simulink model "SimParking"  (R2017b)
settings: Solver=VariableStepAuto  StartTime=0.0  StopTime=1761  RelTol=1e-3
libraries: neural x1111
(part 40 of 60)

== system SimParking/BestNet- 10 delays -100 100 hidden neurons/Layer 3/Delays 1 ==
  "p{3}" : Inport  PortDimensions=100  SampleTime=1
      mask Display: e = 0.06;c1 = [120 230 180]/255;c2 = ([120 230 180]+0)/(256+128);c3 = ([120 230 180]+128)/(256+128);patch([0 1 1 0],[0 0 1 1],c1);patch([0 1 1 1-e 1-e 0+e],[0 0 1 1-e 0+e 0+e],c2);patch([0 0 1 1-e 0+e 0+e],[0 1 1 1-e 1-e 0+e],c3);plot([0 1 1 0 0],[0 0 1 1 0]);
  mux : Mux  Inputs=1
      mask Display: e = 0.06;c1 = [120 150 230]/255;c2 = ([120 150 230]+0)/383;c3 = ([120 150 230]+128)/383;patch([0 1 1 0],[0 0 1 1],c1);patch([0 1 1 1-e 1-e 0+e],[0 0 1 1-e 0+e 0+e],c2);patch([0 0 1 1-e 0+e 0+e],[0 1 1 1-e 1-e 0+e],c3);plot([0 1 1 0 0],[0 0 1 1 0]);disp('Mux')
  "pd{3,2}" : Outport
      mask Display: e = 0.06;c1 = [120 230 180]/255;c2 = ([120 230 180]+0)/(256+128);c3 = ([120 230 180]+128)/(256+128);patch([0 1 1 0],[0 0 1 1],c1);patch([0 1 1 1-e 1-e 0+e],[0 0 1 1-e 0+e 0+e],c2);patch([0 0 1 1-e 0+e 0+e],[0 1 1 1-e 1-e 0+e],c3);plot([0 1 1 0 0],[0 0 1 1 0]);
  wires:
  "p{3}"/1 -> mux/1
  mux/1 -> "pd{3,2}"/1

== system SimParking/BestNet- 10 delays -100 100 hidden neurons/Layer 3/LW{3,2} ==
  "ad{3,2}" : Inport  PortDimensions=100  SampleTime=1
      mask Display: e = 0.06;c1 = [120 230 180]/255;c2 = ([120 230 180]+0)/(256+128);c3 = ([120 230 180]+128)/(256+128);patch([0 1 1 0],[0 0 1 1],c1);patch([0 1 1 1-e 1-e 0+e],[0 0 1 1-e 0+e 0+e],c2);patch([0 0 1 1-e 0+e 0+e],[0 1 1 1-e 1-e 0+e],c3);plot([0 1 1 0 0],[0 0 1 1 0]);
  "IW{3,2}(1,:)'" : Constant  Value=[0.41684320424874876653831279327278025448322296142578125;-0.66619060054073020449294517675298266112804412841796875;0.73244633627706823286729331812239252030849456787109375;-0.77090904802130211237454204820096492767333984375;-0.65642562996155062737813068451941944658756256103515625;0.3805179183622999783409568408387713134288787841796875;-0.6888118551762036911867426169919781386852264404296875;0.7948756177083711182973502218374051153659820556640625;0.93939464145211493129039581617689691483974456787109375;0.21599937852856132547429979240405373275279998779296875;0.308391550957052229531285547636798582971096038818359375;-0.50184938042225202270429917916771955788135528564453125;0.91262609553307438847724597508204169571399688720703125;0.054829250579116528552248155392589978873729705810546875;-0.63302398374616952736460007145069539546966552734375;-0.251138079100727995562891692316043190658092498779296875;-0.001939514422652548197856248179959948174655437469482421875;-0.0248995681144211396251808565693863783963024616241455078125;0.36294553182525157719595654270960949361324310302734375;0.69972765353941712707097622114815749228000640869140625;0.179214291226898747577678250308963470160961151123046875;-0.463920847025235894012240578376804478466510772705078125;0.369260353571986665865978238798561505973339080810546875;-0.76639795402818655656318469482357613742351531982421875;0.1908055213657979809482867494807578623294830322265625;-0.75766996107794770676235884820926003158092498779296875;0.10777304409928968598197940309546538628637790679931640625;0.612941299086788848882179081556387245655059814453125;-0.6959544465686471337306784334941767156124114990234375;0.5753115554941283793510820032679475843906402587890625;0.342991141464252302650805859229876659810543060302734375;-0.6662744617803351143692225377890281379222869873046875;0.1894892352410578462151846679262234829366207122802734375;-0.5022204533702965267849549491074867546558380126953125;0.70623564816158046486549437759094871580600738525390625;-0.89143059355156306633460872035357169806957244873046875;0.1856016942129566082986258379605715163052082061767578125;-0.1499390422372796349836931995014310814440250396728515625;-0.448877117621941768010884743489441461861133575439453125;-0.46907817603243362469811472692526876926422119140625;-1.009712261648737285923971285228617489337921142578125;-0.127129683777713553549659764030366204679012298583984375;0.0271082882605968474021285175012963009066879749298095703125;-0.16083063203455305600897418116801418364048004150390625;0.74753076892948533416216605473891831934452056884765625;-0.019098796952154155348591046958972583524882793426513671875;0.8026380185267061317944126130896620452404022216796875;-0.431133931636676848153655328133027069270610809326171875;-0.1604076740327938510599636856568395160138607025146484375;0.1575254883510431025417375394681585021317005157470703125;-0.72069255985964464361615000598249025642871856689453125;0.7264885215479168767416240370948798954486846923828125;-0.81595174364460187899084075979772023856639862060546875;0.348451729670800680604969556952710263431072235107421875;0.0211956052938375473504439838734469958581030368804931640625;0.120992984761155442097191325956373475492000579833984375;-0.32287042337615190490396344102919101715087890625;-0.38031689040246818844792642266838811337947845458984375;-0.272663150425225875306267653286340646445751190185546875;-0.1941316205827401664141262926932540722191333770751953125;-0.456167815321363800951104394698631949722766876220703125;0.62069030336151065352368050298537127673625946044921875;0.08390607149481459081652445775034721009433269500732421875;0.163239383759437750587295568038825877010822296142578125;-0.21273885412261195337890740120201371610164642333984375;-0.58727754175088808796800776690361090004444122314453125;0.519302834081393438481200064416043460369110107421875;0.895589424860863569932689642882905900478363037109375;-0.892741571184341609068724210374057292938232421875;0.0094276224021251804618959369008734938688576221466064453125 ...(+1715 chars)]
      mask Display: e = 0.06;c1 = [120 150 230]/255;c2 = ([120 150 230]+0)/383;c3 = ([120 150 230]+128)/383;patch([0 1 1 0],[0 0 1 1],c1);patch([0 1 1 1-e 1-e 0+e],[0 0 1 1-e 0+e 0+e],c2);patch([0 0 1 1-e 0+e 0+e],[0 1 1 1-e 1-e 0+e],c3);plot([0 1 1 0 0],[0 0 1 1 0]);disp('weights');
  "IW{3,2}(2,:)'" : Constant  Value=[0.83276048179549244654396034093224443495273590087890625;0.952080926610600730697342441999353468418121337890625;0.55437304436110379501911893385113216936588287353515625;-0.498049896996628216339075834184768609702587127685546875;0.87846289184765280477762416921905241906642913818359375;-0.08363975888338896769180763612894224934279918670654296875;-0.244740578002185793504708044565632008016109466552734375;0.072270072465087265012328998636803589761257171630859375;-0.14696141633061288178652148417313583195209503173828125;0.09751343397330232420916473756733466871082782745361328125;0.12039459153537944435807816034866846166551113128662109375;-0.09107320269378839372453882106128730811178684234619140625;0.18611752915378598771667384426109492778778076171875;-0.1002120169632193802389252823559218086302280426025390625;0.71093278518957514489073901131632737815380096435546875;0.29129601789901815589445277510094456374645233154296875;0.047015580356216717106132563230858067981898784637451171875;0.9438346195589153442284668926731683313846588134765625;0.08747030871269621810082384172346792183816432952880859375;-0.63714099192250162051465167678543366491794586181640625;-0.08685430493060651568892893692463985644280910491943359375;0.291619276402729499242383326418348588049411773681640625;0.144378357746725194399317615534528158605098724365234375;-0.01308257774632117127755481789108671364374458789825439453125;0.1470834172527644423400516870970022864639759063720703125;0.290628216424225926939328701337217353284358978271484375;-0.04400627030965598152079110150225460529327392578125;0.737639956458874923583834970486350357532501220703125;-0.355005641018594386704165799528709612786769866943359375;-0.54014467948711064604339071593130938708782196044921875;-0.32676973764336814110009754585917107760906219482421875;-0.2205672091957241176540804872274748049676418304443359375;-0.2191810573470325262945834765559993684291839599609375;-0.8150047498101973264539310548570938408374786376953125;0.1761038474954243204795290012043551541864871978759765625;0.2593601013148447709255606241640634834766387939453125;-0.9127664176693581765675844508223235607147216796875;-0.5109263846944447351461349171586334705352783203125;-0.79564193970125851596009169952594675123691558837890625;0.273099304739763792948537002303055487573146820068359375;0.11575306736799607920662680271561839617788791656494140625;-0.0897308235222662176067132122625480405986309051513671875;-0.0279566402343247831507877521062255254946649074554443359375;-0.462942098079232089435919306197320111095905303955078125;-0.462906331489028655123973976515117101371288299560546875;-0.337861639674315206161026026165927760303020477294921875;-0.0597844579628253047776098583199200220406055450439453125;0.355840558302590703743106814727070741355419158935546875;0.38049249103025306606440381074207834899425506591796875;0.09920601336196850639215227829481591470539569854736328125;-0.326520932248126227737117233118624426424503326416015625;-0.5188869948383192376439865256543271243572235107421875;-0.6706868969229538013365754522965289652347564697265625;0.1313018089899987417279447754481225274503231048583984375;-0.598907997500010669256198525545187294483184814453125;-0.087051250526162859966206042372505180537700653076171875;0.83797345981939719283815293238149024546146392822265625;-0.57929762290617470288367485409253276884555816650390625;0.1928159026874219084124462142426637001335620880126953125;0.31962269801852516426521333414711989462375640869140625;-0.6646637662275975966252872240147553384304046630859375;-0.29948321827473700640354081770055927336215972900390625;-0.055107534665321693256867519039587932638823986053466796875;-0.1599240894374097943231305407607578672468662261962890625;0.4435983909658898216576972117763943970203399658203125;0.64705868365732788216604376430041156709194183349609375;0.0309419741977244276698311153950271545909345149993896484375;0.74505469760042297711066794363432563841342926025390625;0.479608499136049581945684394668205641210079193115234375 ...(+1737 chars)]
      mask Display: e = 0.06;c1 = [120 150 230]/255;c2 = ([120 150 230]+0)/383;c3 = ([120 150 230]+128)/383;patch([0 1 1 0],[0 0 1 1],c1);patch([0 1 1 1-e 1-e 0+e],[0 0 1 1-e 0+e 0+e],c2);patch([0 0 1 1-e 0+e 0+e],[0 1 1 1-e 1-e 0+e],c3);plot([0 1 1 0 0],[0 0 1 1 0]);disp('weights');
  "IW{3,2}(3,:)'" : Constant  Value=[-0.079867596279532604430784203941584564745426177978515625;0.421026507957778572954765650138142518699169158935546875;-0.00107174772516766881637340080857256907620467245578765869140625;-0.86471162423859804224690606133663095533847808837890625;0.724434206151811199703161037177778780460357666015625;3.4080105290831337327972505590878427028656005859375;0.440951874527029274997147467729519121348857879638671875;0.63292441521918296754023458561277948319911956787109375;-0.019416029383279721776123238896616385318338871002197265625;0.413855818055155477708240141510032117366790771484375;0.43757878674376449179561632263357751071453094482421875;-0.3950488963128966357629678896046243607997894287109375;-0.10068963107221710895355926140837254934012889862060546875;0.316450227424387608987643716318416409194469451904296875;0.4282412652027145494315618634573183953762054443359375;0.1086425974293337148868232588938553817570209503173828125;-0.04779933051416328237959163516279659233987331390380859375;-0.70048238870363344066305444357567466795444488525390625;-0.2130929421796732003979712999353068880736827850341796875;-0.57510791470367494948590092462836764752864837646484375;-0.2245750294346214037677356145650264807045459747314453125;-0.085416833807948899792705788058810867369174957275390625;-0.2730988490222074904778537529637105762958526611328125;0.32671644039610836518505720960092730820178985595703125;0.1099579947694604153962671944100293330848217010498046875;0.1398892909697854458617172213052981533110141754150390625;0.07496086646863094060666554696581442840397357940673828125;-0.316580432772809616803755261571495793759822845458984375;-0.499775643636667654678973349291482008993625640869140625;-0.128520818460897079393845388040062971413135528564453125;0.097562360876206344340033638218301348388195037841796875;0.2086939505948232909116057953724521212279796600341796875;0.1257903689756044995906592021128744818270206451416015625;-0.84357734744596069020872164401225745677947998046875;0.294626622854485209490604802340385504066944122314453125;0.089218291498459001420684444383368827402591705322265625;-0.798440310783131490524056061985902488231658935546875;0.01256074255719878164649916385542383068241178989410400390625;-0.006320676938147508361343085425687604583799839019775390625;-0.139701465391693646633797243339358828961849212646484375;-0.07142656920732425029907375346738263033330440521240234375;0.02604513314789402844695587191381491720676422119140625;-0.052343980255830813153039571261615492403507232666015625;-0.07062540329376136571948308073842781595885753631591796875;-0.1428168474247424601930589460607734508812427520751953125;-0.342809292340396531972857019354705698788166046142578125;0.02392808379663953488591943141727824695408344268798828125;0.1589186323657407751142045526648871600627899169921875;0.346293192334068578031036622633109800517559051513671875;-0.99359866032413879377571674922364763915538787841796875;-1.3643327144396921735136629649787209928035736083984375;-0.43767913286694459795711509286775253713130950927734375;-0.41179903128570061188185036371578462421894073486328125;0.2477217269788194453639107450726442039012908935546875;-0.278054509145230721589570066498708911240100860595703125;-0.0546124447828183201547602720893337391316890716552734375;0.0283251867835226135705628536243239068426191806793212890625;0.81295677933681675941812727614887990057468414306640625;-0.035640932153715422503470477977316477335989475250244140625;0.318792438599860339376590445681358687579631805419921875;0.258180111548097557250258660133113153278827667236328125;0.42630747986609318633810516985249705612659454345703125;0.137146563585003267160544737635063938796520233154296875;-1.0053523193342750463585844045155681669712066650390625;0.342262235453818342012510811400716193020343780517578125;0.1284795972385318896247241582386777736246585845947265625;-0.47979857960265015481837735933368094265460968017578125;-0.8130427661312353837530508826603181660175323486328125;-0.7318141430703548611091946440865285694599151611328125 ...(+1784 chars)]
      mask Display: e = 0.06;c1 = [120 150 230]/255;c2 = ([120 150 230]+0)/383;c3 = ([120 150 230]+128)/383;patch([0 1 1 0],[0 0 1 1],c1);patch([0 1 1 1-e 1-e 0+e],[0 0 1 1-e 0+e 0+e],c2);patch([0 0 1 1-e 0+e 0+e],[0 1 1 1-e 1-e 0+e],c3);plot([0 1 1 0 0],[0 0 1 1 0]);disp('weights');
  Mux : Mux  Inputs=3
      mask Display: e = 0.06;c1 = [120 150 230]/255;c2 = ([120 150 230]+0)/383;c3 = ([120 150 230]+128)/383;patch([0 1 1 0],[0 0 1 1],c1);patch([0 1 1 1-e 1-e 0+e],[0 0 1 1-e 0+e 0+e],c2);patch([0 0 1 1-e 0+e 0+e],[0 1 1 1-e 1-e 0+e],c3);plot([0 1 1 0 0],[0 0 1 1 0]);disp('Mux');
  dotprod1 : neural/Weight Functions/dotprod
  dotprod2 : neural/Weight Functions/dotprod
  dotprod3 : neural/Weight Functions/dotprod
  "lz{3,2}" : Outport
      mask Display: e = 0.06;c1 = [120 230 180]/255;c2 = ([120 230 180]+0)/(256+128);c3 = ([120 230 180]+128)/(256+128);patch([0 1 1 0],[0 0 1 1],c1);patch([0 1 1 1-e 1-e 0+e],[0 0 1 1-e 0+e 0+e],c2);patch([0 0 1 1-e 0+e 0+e],[0 1 1 1-e 1-e 0+e],c3);plot([0 1 1 0 0],[0 0 1 1 0]);
  wires:
  "IW{3,2}(1,:)'"/1 -> dotprod1/1
  "ad{3,2}"/1 -> dotprod1/2, dotprod2/2, dotprod3/2
  dotprod1/1 -> Mux/1
  "IW{3,2}(2,:)'"/1 -> dotprod2/1
  dotprod2/1 -> Mux/2
  "IW{3,2}(3,:)'"/1 -> dotprod3/1
  dotprod3/1 -> Mux/3
  Mux/1 -> "lz{3,2}"/1

== system SimParking/BestNet- 10 delays -100 100 hidden neurons1/Layer 1/Delays 1 ==
  "p{1}" : Inport  PortDimensions=9  SampleTime=1
      mask Display: e = 0.06;c1 = [120 230 180]/255;c2 = ([120 230 180]+0)/(256+128);c3 = ([120 230 180]+128)/(256+128);patch([0 1 1 0],[0 0 1 1],c1);patch([0 1 1 1-e 1-e 0+e],[0 0 1 1-e 0+e 0+e],c2);patch([0 0 1 1-e 0+e 0+e],[0 1 1 1-e 1-e 0+e],c3);plot([0 1 1 0 0],[0 0 1 1 0]);
  Delay 1 : UnitDelay  InitialCondition=pi_input_1_delayed_1
      mask Display: e = 0.06;c1 = [120 150 230]/255;c2 = ([120 150 230]+0)/383;c3 = ([120 150 230]+128)/383;patch([0 1 1 0],[0 0 1 1],c1);patch([0 1 1 1-e 1-e 0+e],[0 0 1 1-e 0+e 0+e],c2);patch([0 0 1 1-e 0+e 0+e],[0 1 1 1-e 1-e 0+e],c3);plot([0 1 1 0 0],[0 0 1 1 0]);disp('D')
  Delay 10 : UnitDelay  InitialCondition=pi_input_1_delayed_10
      mask Display: e = 0.06;c1 = [120 150 230]/255;c2 = ([120 150 230]+0)/383;c3 = ([120 150 230]+128)/383;patch([0 1 1 0],[0 0 1 1],c1);patch([0 1 1 1-e 1-e 0+e],[0 0 1 1-e 0+e 0+e],c2);patch([0 0 1 1-e 0+e 0+e],[0 1 1 1-e 1-e 0+e],c3);plot([0 1 1 0 0],[0 0 1 1 0]);disp('D')
  Delay 2 : UnitDelay  InitialCondition=pi_input_1_delayed_2
      mask Display: e = 0.06;c1 = [120 150 230]/255;c2 = ([120 150 230]+0)/383;c3 = ([120 150 230]+128)/383;patch([0 1 1 0],[0 0 1 1],c1);patch([0 1 1 1-e 1-e 0+e],[0 0 1 1-e 0+e 0+e],c2);patch([0 0 1 1-e 0+e 0+e],[0 1 1 1-e 1-e 0+e],c3);plot([0 1 1 0 0],[0 0 1 1 0]);disp('D')
  Delay 3 : UnitDelay  InitialCondition=pi_input_1_delayed_3
      mask Display: e = 0.06;c1 = [120 150 230]/255;c2 = ([120 150 230]+0)/383;c3 = ([120 150 230]+128)/383;patch([0 1 1 0],[0 0 1 1],c1);patch([0 1 1 1-e 1-e 0+e],[0 0 1 1-e 0+e 0+e],c2);patch([0 0 1 1-e 0+e 0+e],[0 1 1 1-e 1-e 0+e],c3);plot([0 1 1 0 0],[0 0 1 1 0]);disp('D')
  Delay 4 : UnitDelay  InitialCondition=pi_input_1_delayed_4
      mask Display: e = 0.06;c1 = [120 150 230]/255;c2 = ([120 150 230]+0)/383;c3 = ([120 150 230]+128)/383;patch([0 1 1 0],[0 0 1 1],c1);patch([0 1 1 1-e 1-e 0+e],[0 0 1 1-e 0+e 0+e],c2);patch([0 0 1 1-e 0+e 0+e],[0 1 1 1-e 1-e 0+e],c3);plot([0 1 1 0 0],[0 0 1 1 0]);disp('D')
  Delay 5 : UnitDelay  InitialCondition=pi_input_1_delayed_5
      mask Display: e = 0.06;c1 = [120 150 230]/255;c2 = ([120 150 230]+0)/383;c3 = ([120 150 230]+128)/383;patch([0 1 1 0],[0 0 1 1],c1);patch([0 1 1 1-e 1-e 0+e],[0 0 1 1-e 0+e 0+e],c2);patch([0 0 1 1-e 0+e 0+e],[0 1 1 1-e 1-e 0+e],c3);plot([0 1 1 0 0],[0 0 1 1 0]);disp('D')
  Delay 6 : UnitDelay  InitialCondition=pi_input_1_delayed_6
      mask Display: e = 0.06;c1 = [120 150 230]/255;c2 = ([120 150 230]+0)/383;c3 = ([120 150 230]+128)/383;patch([0 1 1 0],[0 0 1 1],c1);patch([0 1 1 1-e 1-e 0+e],[0 0 1 1-e 0+e 0+e],c2);patch([0 0 1 1-e 0+e 0+e],[0 1 1 1-e 1-e 0+e],c3);plot([0 1 1 0 0],[0 0 1 1 0]);disp('D')
  Delay 7 : UnitDelay  InitialCondition=pi_input_1_delayed_7
      mask Display: e = 0.06;c1 = [120 150 230]/255;c2 = ([120 150 230]+0)/383;c3 = ([120 150 230]+128)/383;patch([0 1 1 0],[0 0 1 1],c1);patch([0 1 1 1-e 1-e 0+e],[0 0 1 1-e 0+e 0+e],c2);patch([0 0 1 1-e 0+e 0+e],[0 1 1 1-e 1-e 0+e],c3);plot([0 1 1 0 0],[0 0 1 1 0]);disp('D')
  Delay 8 : UnitDelay  InitialCondition=pi_input_1_delayed_8
      mask Display: e = 0.06;c1 = [120 150 230]/255;c2 = ([120 150 230]+0)/383;c3 = ([120 150 230]+128)/383;patch([0 1 1 0],[0 0 1 1],c1);patch([0 1 1 1-e 1-e 0+e],[0 0 1 1-e 0+e 0+e],c2);patch([0 0 1 1-e 0+e 0+e],[0 1 1 1-e 1-e 0+e],c3);plot([0 1 1 0 0],[0 0 1 1 0]);disp('D')
  Delay 9 : UnitDelay  InitialCondition=pi_input_1_delayed_9
      mask Display: e = 0.06;c1 = [120 150 230]/255;c2 = ([120 150 230]+0)/383;c3 = ([120 150 230]+128)/383;patch([0 1 1 0],[0 0 1 1],c1);patch([0 1 1 1-e 1-e 0+e],[0 0 1 1-e 0+e 0+e],c2);patch([0 0 1 1-e 0+e 0+e],[0 1 1 1-e 1-e 0+e],c3);plot([0 1 1 0 0],[0 0 1 1 0]);disp('D')
  mux : Mux  Inputs=10
      mask Display: e = 0.06;c1 = [120 150 230]/255;c2 = ([120 150 230]+0)/383;c3 = ([120 150 230]+128)/383;patch([0 1 1 0],[0 0 1 1],c1);patch([0 1 1 1-e 1-e 0+e],[0 0 1 1-e 0+e 0+e],c2);patch([0 0 1 1-e 0+e 0+e],[0 1 1 1-e 1-e 0+e],c3);plot([0 1 1 0 0],[0 0 1 1 0]);disp('Mux')
  "pd{1,1}" : Outport
      mask Display: e = 0.06;c1 = [120 230 180]/255;c2 = ([120 230 180]+0)/(256+128);c3 = ([120 230 180]+128)/(256+128);patch([0 1 1 0],[0 0 1 1],c1);patch([0 1 1 1-e 1-e 0+e],[0 0 1 1-e 0+e 0+e],c2);patch([0 0 1 1-e 0+e 0+e],[0 1 1 1-e 1-e 0+e],c3);plot([0 1 1 0 0],[0 0 1 1 0]);
  wires:
  "p{1}"/1 -> Delay 1/1
  Delay 1/1 -> Delay 2/1, mux/1
  Delay 2/1 -> Delay 3/1, mux/2
  Delay 3/1 -> Delay 4/1, mux/3
  Delay 4/1 -> Delay 5/1, mux/4
  Delay 5/1 -> Delay 6/1, mux/5
  Delay 6/1 -> Delay 7/1, mux/6
  Delay 7/1 -> Delay 8/1, mux/7
  Delay 8/1 -> Delay 9/1, mux/8
  Delay 9/1 -> Delay 10/1, mux/9
  Delay 10/1 -> mux/10
  mux/1 -> "pd{1,1}"/1
